simulink subsystem "coil_led_control"  (R2024b)
settings: Solver=VariableStepAuto  StartTime=0.0  StopTime=10.0  RelTol=1e-3
undefined symbols (not defined in the file or in its folder): TempStg_High, TempStg_Low, TempStg_Med
settings Model: Creator=developer  LastModifiedBy=developer

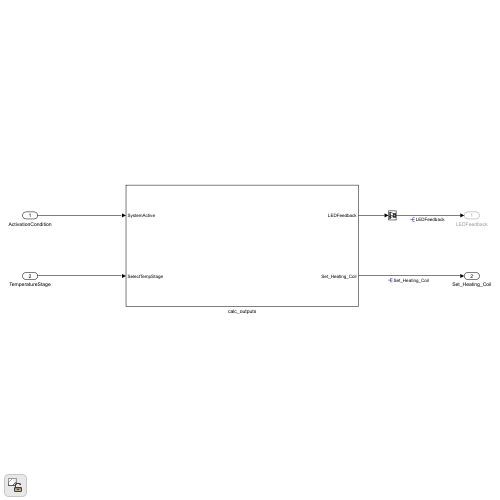
[thumbnail: Simulink's stored preview of the top-level diagram]
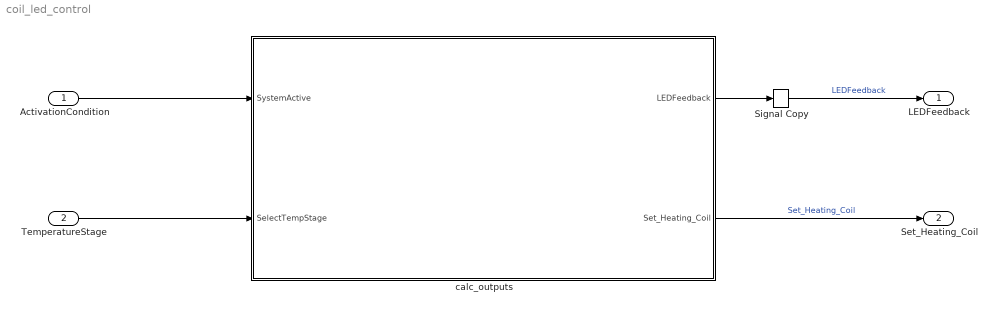
== system coil_led_control ==
  ActivationCondition : Inport
  TemperatureStage : Inport  Port=2
  Signal Copy : SignalConversion  OverrideOpt=off
  calc_outputs : Subsystem
  LEDFeedback : Outport
      settings: EnsureOutportIsVirtual=on
  Set_Heating_Coil : Outport  Port=2
  wires:
  TemperatureStage/1 -> calc_outputs/2(SelectTempStage)
  calc_outputs/1(LEDFeedback) -> Signal Copy/1
  calc_outputs/2(Set_Heating_Coil) -> Set_Heating_Coil/1  "Set_Heating_Coil"
  Signal Copy/1 -> LEDFeedback/1  "LEDFeedback"
  ActivationCondition/1 -> calc_outputs/1(SystemActive)

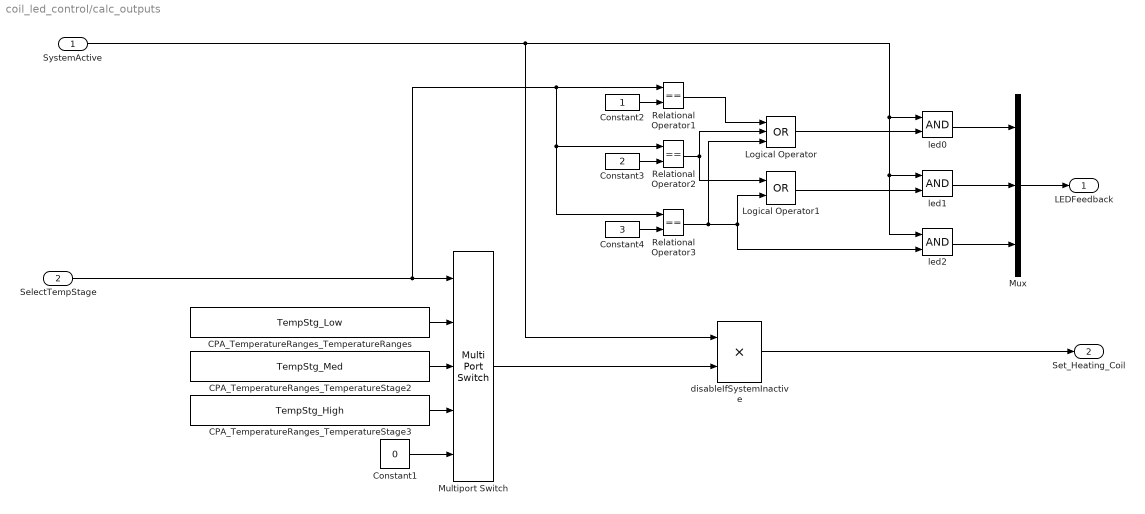
== system coil_led_control/calc_outputs ==
  SystemActive : Inport
  SelectTempStage : Inport  Port=2
  CPA_TemperatureRanges_TemperatureRanges : Constant  Value=TempStg_Low
  CPA_TemperatureRanges_TemperatureStage2 : Constant  Value=TempStg_Med
  CPA_TemperatureRanges_TemperatureStage3 : Constant  Value=TempStg_High
  Constant1 : Constant  Value=0
  Constant2 : Constant  OutDataTypeStr=Inherit: Inherit via back propagation
  Constant3 : Constant  Value=2  OutDataTypeStr=Inherit: Inherit via back propagation
  Constant4 : Constant  Value=3  OutDataTypeStr=Inherit: Inherit via back propagation
  Logical Operator : Logic  Operator=OR  Inputs=3  AllPortsSameDT=off  OutDataTypeStr=boolean
  Logical Operator1 : Logic  Operator=OR  AllPortsSameDT=off  OutDataTypeStr=boolean
  Multiport Switch : MultiPortSwitch  DataPortIndices={0,1,2,3}  DataPortForDefault=Additional data port  DiagnosticForDefault=None  OutDataTypeStr=uint8  SaturateOnIntegerOverflow=off  InputSameDT=off
  Mux : Mux  Inputs=3
  Relational Operator1 : RelationalOperator  Operator===  OutDataTypeStr=boolean  RndMeth=Simplest  InputSameDT=off
  Relational Operator2 : RelationalOperator  Operator===  OutDataTypeStr=boolean  RndMeth=Simplest  InputSameDT=off
  Relational Operator3 : RelationalOperator  Operator===  OutDataTypeStr=boolean  RndMeth=Simplest  InputSameDT=off
  disableIfSystemInactive : Product
  led0 : Logic  AllPortsSameDT=off  OutDataTypeStr=boolean
  led1 : Logic  AllPortsSameDT=off  OutDataTypeStr=boolean
  led2 : Logic  AllPortsSameDT=off  OutDataTypeStr=boolean
  LEDFeedback : Outport
  Set_Heating_Coil : Outport  Port=2
  wires:
  led0/1 -> Mux/1
  led2/1 -> Mux/3
  led1/1 -> Mux/2
  Multiport Switch/1 -> disableIfSystemInactive/2
  SystemActive/1 -> led0/1, led1/1, led2/1, disableIfSystemInactive/1
  disableIfSystemInactive/1 -> Set_Heating_Coil/1
  Logical Operator1/1 -> led1/2
  Logical Operator/1 -> led0/2
  CPA_TemperatureRanges_TemperatureRanges/1 -> Multiport Switch/2
  CPA_TemperatureRanges_TemperatureStage3/1 -> Multiport Switch/4
  Constant1/1 -> Multiport Switch/5
  Relational Operator3/1 -> Logical Operator1/2, led2/2, Logical Operator/3
  Constant3/1 -> Relational Operator2/2
  Relational Operator1/1 -> Logical Operator/1
  Relational Operator2/1 -> Logical Operator/2, Logical Operator1/1
  CPA_TemperatureRanges_TemperatureStage2/1 -> Multiport Switch/3
  Mux/1 -> LEDFeedback/1
  Constant4/1 -> Relational Operator3/2
  Constant2/1 -> Relational Operator1/2
  SelectTempStage/1 -> Multiport Switch/1, Relational Operator1/1, Relational Operator2/1, Relational Operator3/1
